simulink model "Octacopter_Model"  (R2025b)
settings: Solver=VariableStepAuto  StartTime=0.0  StopTime=10  RelTol=1e-3
values from neighbouring files (symbols this model uses):
  Alt = 600    [Octa_Initialise.m]
  c = -500    [Octa_Initialise.m]
  Drag_on = 1    [Octa_Initialise.m]
  g = 9.81    [Octa_Initialise.m]
  I = [I_xx, I_xy, I_xz; I_xy, I_yy, I_yz; I_xz, I_yz, I_zz]    [Octa_Initialise.m]
  I_xx = 0.35    [Octa_Initialise.m]
  I_yy = 0.35    [Octa_Initialise.m]
  I_zz = 0.67    [Octa_Initialise.m]
  k = 6500    [Octa_Initialise.m]
  k_D = [0.05, 0.05, 0.15]    [Octa_Initialise.m]
  k_q = (Cp*Rho*(D)^5)/(8*(pi)^3)    (= 1.08765022525e-07)    [Octa_Initialise.m]
  l_arm1 = [l*cosd(0) l*sind(0) 0]    [Octa_Initialise.m]
  l_arm2 = [l*cosd(-45) l*sind(-45) 0]    [Octa_Initialise.m]
  l_arm3 = [l*cosd(-90) l*sind(-90) 0]    [Octa_Initialise.m]
  l_arm4 = [l*cosd(-135) l*sind(-135) 0]    [Octa_Initialise.m]
  l_arm5 = [l*cosd(-180) l*sind(-180) 0]    [Octa_Initialise.m]
  l_arm6 = [l*cosd(135) l*sind(135) 0]    [Octa_Initialise.m]
  l_arm7 = [l*cosd(90) l*sind(90) 0]    [Octa_Initialise.m]
  l_arm8 = [l*cosd(45) l*sind(45) 0]    [Octa_Initialise.m]
  m = 6.71    [Octa_Initialise.m]
  M1_set_phi = 0    [Octa_Initialise.m]
  M1_set_theta = 0    [Octa_Initialise.m]
  M2_set_phi = 0    [Octa_Initialise.m]
  M2_set_theta = 0    [Octa_Initialise.m]
  M3_set_phi = 0    [Octa_Initialise.m]
  M3_set_theta = 0    [Octa_Initialise.m]
  M4_set_phi = 0    [Octa_Initialise.m]
  M4_set_theta = 0    [Octa_Initialise.m]
  M5_set_phi = 0    [Octa_Initialise.m]
  M5_set_theta = 0    [Octa_Initialise.m]
  M6_set_phi = 0    [Octa_Initialise.m]
  M6_set_theta = 0    [Octa_Initialise.m]
  M7_set_phi = 0    [Octa_Initialise.m]
  M7_set_theta = 0    [Octa_Initialise.m]
  M8_set_phi = 0    [Octa_Initialise.m]
  M8_set_theta = 0    [Octa_Initialise.m]
  p_dot_dot_0 = 0    [Octa_Initialise.m]
  phi_dot_0 = phi_theta_psi_dot_0(1)    [Octa_Initialise.m]
  phi_lower = deg2rad(-180)    [Octa_Initialise.m]
  phi_upper = deg2rad(180)    [Octa_Initialise.m]
  psi_dot_0 = phi_theta_psi_dot_0(3)    [Octa_Initialise.m]
  q_dot_dot_0 = 0    [Octa_Initialise.m]
  r_dot_dot_0 = 0    [Octa_Initialise.m]
  rpm2rad_s = pi/30    (= 0.10471975512)    [Octa_Initialise.m]
  RPM_max = 17668    [Octa_Initialise.m]    (also in Thrust_Plots.m = 15000)
  RPM_min = 0    [Octa_Initialise.m]    (also in Thrust_Plots.m)
  Tau_ESC1 = 0.15    [Octa_Initialise.m]
  Tau_ESC2 = 0.15    [Octa_Initialise.m]
  Tau_ESC3 = 0.15    [Octa_Initialise.m]
  Tau_ESC4 = 0.15    [Octa_Initialise.m]
  Tau_ESC5 = 0.15    [Octa_Initialise.m]
  Tau_ESC6 = 0.15    [Octa_Initialise.m]
  Tau_ESC7 = 0.15    [Octa_Initialise.m]
  Tau_ESC8 = 0.15    [Octa_Initialise.m]
  theta_dot_0 = phi_theta_psi_dot_0(2)    [Octa_Initialise.m]
  theta_lower = deg2rad(-90)    [Octa_Initialise.m]
  theta_upper = deg2rad(90)    [Octa_Initialise.m]
  Thrust_max = 20    [Octa_Initialise.m]
  thrustData = load('Cine66 Thrust Params.mat')    [Thrust_Plots.m]
  u_0 = u_v_w_0(1)    [Octa_Initialise.m]
  u_dot_0 = 0    [Octa_Initialise.m]
  v_0 = u_v_w_0(2)    [Octa_Initialise.m]
  v_dot_0 = 0    [Octa_Initialise.m]
  w1_0 = 0    [Octa_Initialise.m]
  w2_0 = 0    [Octa_Initialise.m]
  w3_0 = 0    [Octa_Initialise.m]
  w4_0 = 0    [Octa_Initialise.m]
  w5_0 = 0    [Octa_Initialise.m]
  w6_0 = 0    [Octa_Initialise.m]
  w7_0 = 0    [Octa_Initialise.m]
  w8_0 = 0    [Octa_Initialise.m]
  w_0 = u_v_w_0(3)    [Octa_Initialise.m]
  w_d_1 = -1    [Octa_Initialise.m]
  w_d_2 = +1.    (= 1)    [Octa_Initialise.m]
  w_d_3 = -1    [Octa_Initialise.m]
  w_d_4 = +1    (= 1)    [Octa_Initialise.m]
  w_d_5 = -1    [Octa_Initialise.m]
  w_d_6 = +1    (= 1)    [Octa_Initialise.m]
  w_d_7 = -1    [Octa_Initialise.m]
  w_d_8 = +1    (= 1)    [Octa_Initialise.m]
  w_dot_0 = 0    [Octa_Initialise.m]
undefined symbols (not defined in the file or in its folder): DiscIntNeverNeededParam
libraries: matrix_library x10, simulink x3, px4uORBlib x2, px4Sensorslib x2, sharedtransform x1, aerolibutil x1, px4Peripheralslib x1
(part 2 of 2)

== matlab function Octacopter_Model/Plant/Force & Moments/Thrust Forces and Moments/MATLAB Function10 ==
  data: phi input; theta input; T_mot_in input; T_b_out output
function T_b_out = fcn(phi, theta, T_mot_in)
%#codegen

%       phi    : phi angle (phi) about the body x-axis (radians)
%       theta   : theta angle (theta) about the intermediate y-axis (radians)
%       psi     : psi angle (psi) about the inertial z-axis (radians)
%
%   Note: This function assumes a standard Z-Y-X (psi-theta-phi) rotation
%   sequence to construct the rotation matrix R_i_b.

    % --- 1. Define the elementary rotation matrices ---
    
    % phi Rotation about x-axis (R_x(phi))
    Rx = [1,           0,          0;
          0,    cos(phi), -sin(phi);
          0,    sin(phi),  cos(phi)];
      
    % theta Rotation about y-axis (R_y(theta))
    Ry = [cos(theta),  0, sin(theta);
                 0,  1,          0;
         -sin(theta),  0, cos(theta)];
     

    % --- 2. Construct the full Rotation Matrix (DCM) ---
    % R_i_b = R_x(phi) * R_y(theta) 
    % This transforms a vector from  Inertial (i) to Body (b) frame.
    R_i_b = Rx * Ry;
    
    % --- 3. Apply the transformation ---
    T_b_out = R_i_b * T_mot_in;

== matlab function Octacopter_Model/Plant/Force & Moments/Thrust Forces and Moments/MATLAB Function11 ==
  data: phi input; theta input; T_mot_in input; T_b_out output
function T_b_out = fcn(phi, theta, T_mot_in)
%#codegen

%       phi    : phi angle (phi) about the body x-axis (radians)
%       theta   : theta angle (theta) about the intermediate y-axis (radians)
%       psi     : psi angle (psi) about the inertial z-axis (radians)
%
%   Note: This function assumes a standard Z-Y-X (psi-theta-phi) rotation
%   sequence to construct the rotation matrix R_i_b.

    % --- 1. Define the elementary rotation matrices ---
    
    % phi Rotation about x-axis (R_x(phi))
    Rx = [1,           0,          0;
          0,    cos(phi), -sin(phi);
          0,    sin(phi),  cos(phi)];
      
    % theta Rotation about y-axis (R_y(theta))
    Ry = [cos(theta),  0, sin(theta);
                 0,  1,          0;
         -sin(theta),  0, cos(theta)];
     

    % --- 2. Construct the full Rotation Matrix (DCM) ---
    % R_i_b = R_x(phi) * R_y(theta) 
    % This transforms a vector from  Inertial (i) to Body (b) frame.
    R_i_b = Rx * Ry;
    
    % --- 3. Apply the transformation ---
    T_b_out = R_i_b * T_mot_in;

== matlab function Octacopter_Model/Plant/Force & Moments/Thrust Forces and Moments/MATLAB Function12 ==
  data: phi input; theta input; T_mot_in input; T_b_out output
function T_b_out = fcn(phi, theta, T_mot_in)
%#codegen

%       phi    : phi angle (phi) about the body x-axis (radians)
%       theta   : theta angle (theta) about the intermediate y-axis (radians)
%       psi     : psi angle (psi) about the inertial z-axis (radians)
%
%   Note: This function assumes a standard Z-Y-X (psi-theta-phi) rotation
%   sequence to construct the rotation matrix R_i_b.

    % --- 1. Define the elementary rotation matrices ---
    
    % phi Rotation about x-axis (R_x(phi))
    Rx = [1,           0,          0;
          0,    cos(phi), -sin(phi);
          0,    sin(phi),  cos(phi)];
      
    % theta Rotation about y-axis (R_y(theta))
    Ry = [cos(theta),  0, sin(theta);
                 0,  1,          0;
         -sin(theta),  0, cos(theta)];
     

    % --- 2. Construct the full Rotation Matrix (DCM) ---
    % R_i_b = R_x(phi) * R_y(theta) 
    % This transforms a vector from  Inertial (i) to Body (b) frame.
    R_i_b = Rx * Ry;
    
    % --- 3. Apply the transformation ---
    T_b_out = R_i_b * T_mot_in;

== matlab function Octacopter_Model/Subsystem/Estimation1/MATLAB Function ==
  data: yaw_w input; yaw_u output
function yaw_u = unwrap_yaw(yaw_w)
% yaw_w: wrapped yaw [rad], typically in [-pi, pi]
% yaw_u: continuous yaw [rad]

persistent yaw_prev yaw_accum initialized

if isempty(initialized)
    yaw_prev = yaw_w;
    yaw_accum = yaw_w;
    initialized = true;
end

dyaw = yaw_w - yaw_prev;

% wrap increment to [-pi, pi]
dyaw = mod(dyaw + pi, 2*pi) - pi;

yaw_accum = yaw_accum + dyaw;
yaw_prev = yaw_w;

yaw_u = yaw_accum;

== matlab function Octacopter_Model/Plant/EOM/MATLAB Function ==
  data: phi input; PhiThetaPsi_dot output; theta input; pqr_dot input
function PhiThetaPsi_dot = fcn(phi, theta, pqr_dot)
%#codegen

Rot = [
    1 sind(phi)*tan(theta) cosd(phi)*tan(theta);
    0 cosd(theta) -sind(phi);
    0 sin(phi)*secd(theta) cosd(phi)*secd(theta)
    ];

PhiThetaPsi_dot = Rot*pqr_dot;

== matlab function Octacopter_Model/Plant/EOM/MATLAB Function1 ==
  data: F_b_net input; phi input; xyz_dot_dot output; theta input; psi input
function xyz_dot_dot = fcn(F_b_net, phi, theta, psi)
%#codegen
% BODY_TO_INERTIAL Converts a vector from the Body Frame to the Inertial Frame.
%
%   v_inertial = BODY_TO_INERTIAL(v_body, phi, theta, psi)
%
%   Inputs:
%       v_body  : 3x1 vector in the Body Frame (e.g., [x_b; y_b; z_b])
%       phi    : phi angle (phi) about the body x-axis (radians)
%       theta   : theta angle (theta) about the intermediate y-axis (radians)
%       psi     : psi angle (psi) about the inertial z-axis (radians)
%
%   Output:
%       v_inertial : 3x1 vector in the Inertial Frame (e.g., [x_i; y_i; z_i])
%
%   Note: This function assumes a standard Z-Y-X (psi-theta-phi) rotation
%   sequence to construct the rotation matrix R_i_b.

    % --- 1. Define the elementary rotation matrices ---
    
    % phi Rotation about x-axis (R_x(phi))
    Rx = [1,           0,          0;
          0,    cos(phi), -sin(phi);
          0,    sin(phi),  cos(phi)];
      
    % theta Rotation about y-axis (R_y(theta))
    Ry = [cos(theta),  0, sin(theta);
                 0,  1,          0;
         -sin(theta),  0, cos(theta)];
     
    % psi Rotation about z-axis (R_z(psi))
    Rz = [cos(psi), -sin(psi), 0;
          sin(psi),  cos(psi), 0;
               0,         0, 1];
    
    % --- 2. Construct the full Rotation Matrix (DCM) ---
    % R_i_b = R_x(phi) * R_y(theta) * R_z(psi)
    % This transforms a vector from Body (b) to Inertial (i) frame.
    R_i_b = Rz * Ry * Rx;
    
    % --- 3. Apply the transformation ---
    xyz_dot_dot = R_i_b * F_b_net;

== matlab function Octacopter_Model/Plant/EOM/MATLAB Function2 ==
  data: xyz_dot input; phi input; theta input; psi input; uvw output
function uvw = fcn( xyz_dot,phi, theta, psi)
%#codegen

%       phi    : phi angle (phi) about the body x-axis (radians)
%       theta   : theta angle (theta) about the intermediate y-axis (radians)
%       psi     : psi angle (psi) about the inertial z-axis (radians)
%
%   Note: This function assumes a standard Z-Y-X (psi-theta-phi) rotation
%   sequence to construct the rotation matrix R_i_b.

    % --- 1. Define the elementary rotation matrices ---
    
    % phi Rotation about x-axis (R_x(phi))
    Rx = [1,           0,          0;
          0,    cos(phi), -sin(phi);
          0,    sin(phi),  cos(phi)];
      
    % theta Rotation about y-axis (R_y(theta))
    Ry = [cos(theta),  0, sin(theta);
                 0,  1,          0;
         -sin(theta),  0, cos(theta)];
     
    % psi Rotation about z-axis (R_z(psi))
    Rz = [cos(psi), -sin(psi), 0;
          sin(psi),  cos(psi), 0;
               0,         0, 1];
    
    % --- 2. Construct the full Rotation Matrix (DCM) ---
    % R_i_b = R_x(phi) * R_y(theta) * R_z(psi)
    % This transforms a vector from  Inertial (i) to Body (b) frame.
    R_i_b = Rx * Ry * Rz;
    
    % --- 3. Apply the transformation ---
    uvw = R_i_b * xyz_dot;

== matlab function Octacopter_Model/Subsystem/motor mxer1 ==
  data: Roll input; M1 output; Pitch input; Thrust input; Yaw input; M2 output; M3 output; M4 output; M5 output; M6 output; M7 output; M8 output
function [M1, M2, M3, M4, M5, M6, M7, M8] = motor_mixer(Roll, Pitch, Thrust, Yaw)
% This function calculates motor commands for the 8-motor "plus" 
% configuration shown in your image.
%
% Inputs (assumed):
%   Roll, Pitch, Yaw: -1.0 to +1.0 control inputs
%   Thrust:             0.0 to 1.0 base throttle

% --- Configuration ---
idle_PWM = uint16(1000);
max_motor_val = single(1.0); % Max normalized output
min_motor_val = single(0.0); % Min normalized output

% This scaling method is from your example. It scales the control 
% inputs by the thrust level. You may need to tune the '4.0'
% denominator for best performance.
control_scale = Thrust / single(4.0);

% --- Mixer Logic ---
% Calculate normalized motor values (0.0 to 1.0 range) based on the diagram.
% We use single() to ensure floating-point math, as in your example.

% M1 (Front, CCW): -Pitch, +Yaw
m1_norm = ( ( -Pitch + Yaw ) * control_scale + Thrust );

% M2 (Back, CCW): +Pitch, +Yaw
m2_norm = ( (  Pitch + Yaw ) * control_scale + Thrust );

% M3 (Front-Right, CW): -Pitch, -Roll, -Yaw
m3_norm = ( ( -Pitch - Roll - Yaw ) * control_scale + Thrust );

% M4 (Back-Right, CW): +Pitch, -Roll, -Yaw
m4_norm = ( (  Pitch - Roll - Yaw ) * control_scale + Thrust );

% M5 (Front-Left, CW): -Pitch, +Roll, -Yaw
m5_norm = ( ( -Pitch + Roll - Yaw ) * control_scale + Thrust );

% M6 (Back-Left, CW): +Pitch, +Roll, -Yaw
m6_norm = ( (  Pitch + Roll - Yaw ) * control_scale + Thrust );

% M7 (Left, CCW): +Roll, +Yaw
m7_norm = ( (  Roll + Yaw ) * control_scale + Thrust );

% M8 (Right, CCW): -Roll, +Yaw
m8_norm = ( ( -Roll + Yaw ) * control_scale + Thrust );


% --- Output Scaling and Clamping ---
% It's CRITICAL to clamp (saturate) the motor commands between 0.0 and 1.0
% to prevent errors and ensure motor outputs are valid.
motors_norm = [m1_norm, m2_norm, m3_norm, m4_norm, m5_norm, m6_norm, m7_norm, m8_norm];
motors_norm = min(max(motors_norm, min_motor_val), max_motor_val);

% Convert normalized values (0.0-1.0) to PWM (1000-2000)
M1 = uint16(motors_norm(1) * single(1000)) + idle_PWM;
M2 = uint16(motors_norm(2) * single(1000)) + idle_PWM;
M3 = uint16(motors_norm(3) * single(1000)) + idle_PWM;
M4 = uint16(motors_norm(4) * single(1000)) + idle_PWM;
M5 = uint16(motors_norm(5) * single(1000)) + idle_PWM;
M6 = uint16(motors_norm(6) * single(1000)) + idle_PWM;
M7 = uint16(motors_norm(7) * single(1000)) + idle_PWM;
M8 = uint16(motors_norm(8) * single(1000)) + idle_PWM;

end

== matlab function Octacopter_Model/Plant/Force & Moments/Other Forces/Landing Gear Force/MATLAB Function3 ==
  data: phi input; theta input; psi input; F_b_Ldg output; F_ldg input
function F_b_Ldg = fcn(phi, theta, psi, F_ldg)
%#codegen

%       phi    : phi angle (phi) about the body x-axis (radians)
%       theta   : theta angle (theta) about the intermediate y-axis (radians)
%       psi     : psi angle (psi) about the inertial z-axis (radians)
%
%   Note: This function assumes a standard Z-Y-X (psi-theta-phi) rotation
%   sequence to construct the rotation matrix R_i_b.

    % --- 1. Define the elementary rotation matrices ---
    
    % phi Rotation about x-axis (R_x(phi))
    Rx = [1,           0,          0;
          0,    cos(phi), -sin(phi);
          0,    sin(phi),  cos(phi)];
      
    % theta Rotation about y-axis (R_y(theta))
    Ry = [cos(theta),  0, sin(theta);
                 0,  1,          0;
         -sin(theta),  0, cos(theta)];
     
    % psi Rotation about z-axis (R_z(psi))
    Rz = [cos(psi), -sin(psi), 0;
          sin(psi),  cos(psi), 0;
               0,         0, 1];
    
    % --- 2. Construct the full Rotation Matrix (DCM) ---
    % R_i_b = R_x(phi) * R_y(theta) * R_z(psi)
    % This transforms a vector from  Inertial (i) to Body (b) frame.
    R_i_b = Rx * Ry * Rz;
    
    % --- 3. Apply the transformation ---
    F_b_Ldg = R_i_b * F_ldg;

== matlab function Octacopter_Model/Plant/Force & Moments/Other Forces/Inertial 2 Body ==
  data: phi input; theta input; psi input; F_D_b output; F_D_i input
function F_D_b = fcn(phi, theta, psi, F_D_i)
%#codegen

%       phi    : phi angle (phi) about the body x-axis (radians)
%       theta   : theta angle (theta) about the intermediate y-axis (radians)
%       psi     : psi angle (psi) about the inertial z-axis (radians)
%
%   Note: This function assumes a standard Z-Y-X (psi-theta-phi) rotation
%   sequence to construct the rotation matrix R_i_b.

    % --- 1. Define the elementary rotation matrices ---
    
    % phi Rotation about x-axis (R_x(phi))
    Rx = [1,           0,          0;
          0,    cos(phi), -sin(phi);
          0,    sin(phi),  cos(phi)];
      
    % theta Rotation about y-axis (R_y(theta))
    Ry = [cos(theta),  0, sin(theta);
                 0,  1,          0;
         -sin(theta),  0, cos(theta)];
     
    % psi Rotation about z-axis (R_z(psi))
    Rz = [cos(psi), -sin(psi), 0;
          sin(psi),  cos(psi), 0;
               0,         0, 1];
    
    % --- 2. Construct the full Rotation Matrix (DCM) ---
    % R_i_b = R_x(phi) * R_y(theta) * R_z(psi)
    % This transforms a vector from  Inertial (i) to Body (b) frame.
    R_i_b = Rx * Ry * Rz;
    
    % --- 3. Apply the transformation ---
    F_D_b = R_i_b*F_D_i;

== matlab function Octacopter_Model/Plant/Force & Moments/Other Forces/Gravity Force ==
  data: phi input; theta input; psi input; F_g output; m_g input
function F_g = fcn(phi, theta, psi, m_g)
%#codegen

%       phi    : phi angle (phi) about the body x-axis (radians)
%       theta   : theta angle (theta) about the intermediate y-axis (radians)
%       psi     : psi angle (psi) about the inertial z-axis (radians)
%
%   Note: This function assumes a standard Z-Y-X (psi-theta-phi) rotation
%   sequence to construct the rotation matrix R_i_b.

    % --- 1. Define the elementary rotation matrices ---
    
    % phi Rotation about x-axis (R_x(phi))
    Rx = [1,           0,          0;
          0,    cos(phi), -sin(phi);
          0,    sin(phi),  cos(phi)];
      
    % theta Rotation about y-axis (R_y(theta))
    Ry = [cos(theta),  0, sin(theta);
                 0,  1,          0;
         -sin(theta),  0, cos(theta)];
     
    % psi Rotation about z-axis (R_z(psi))
    Rz = [cos(psi), -sin(psi), 0;
          sin(psi),  cos(psi), 0;
               0,         0, 1];
    
    % --- 2. Construct the full Rotation Matrix (DCM) ---
    % R_i_b = R_x(phi) * R_y(theta) * R_z(psi)
    % This transforms a vector from  Inertial (i) to Body (b) frame.
    R_i_b = Rx * Ry * Rz;
    
    % --- 3. Apply the transformation ---
    F_g = R_i_b * [0 0 -m_g]';

== matlab function Octacopter_Model/Plant/Force & Moments/Other Forces/Drag Force ==
  data: F_D output; u input; v input; w input; k_D input
function F_D = fcn(u, v, w, k_D)
%#codegen
    
    k_d_x = k_D(1);
    k_d_y = k_D(2);
    k_d_z = k_D(3);
    
    F_D_x = u*u*k_d_x;
    F_D_y = v*v*k_d_y;
    F_D_z = w*w*k_d_z;

    % --- 3. Apply the transformation ---
    F_D = [F_D_x; F_D_y; F_D_z;];

== matlab function Octacopter_Model/Plant/Force & Moments/Thrust Forces and Moments/MATLAB Function9 ==
  data: phi input; theta input; T_mot_in input; T_b_out output
function T_b_out = fcn(phi, theta, T_mot_in)
%#codegen

%       phi    : phi angle (phi) about the body x-axis (radians)
%       theta   : theta angle (theta) about the intermediate y-axis (radians)
%       psi     : psi angle (psi) about the inertial z-axis (radians)
%
%   Note: This function assumes a standard Z-Y-X (psi-theta-phi) rotation
%   sequence to construct the rotation matrix R_i_b.

    % --- 1. Define the elementary rotation matrices ---
    
    % phi Rotation about x-axis (R_x(phi))
    Rx = [1,           0,          0;
          0,    cos(phi), -sin(phi);
          0,    sin(phi),  cos(phi)];
      
    % theta Rotation about y-axis (R_y(theta))
    Ry = [cos(theta),  0, sin(theta);
                 0,  1,          0;
         -sin(theta),  0, cos(theta)];
     

    % --- 2. Construct the full Rotation Matrix (DCM) ---
    % R_i_b = R_x(phi) * R_y(theta) 
    % This transforms a vector from  Inertial (i) to Body (b) frame.
    R_i_b = Rx * Ry;
    
    % --- 3. Apply the transformation ---
    T_b_out = R_i_b * T_mot_in;

== matlab function Octacopter_Model/Plant/Force & Moments/Thrust Forces and Moments/MATLAB Function5 ==
  data: phi input; theta input; T_mot_in input; T_b_out output
function T_b_out = fcn(phi, theta, T_mot_in)
%#codegen

%       phi    : phi angle (phi) about the body x-axis (radians)
%       theta   : theta angle (theta) about the intermediate y-axis (radians)
%       psi     : psi angle (psi) about the inertial z-axis (radians)
%
%   Note: This function assumes a standard Z-Y-X (psi-theta-phi) rotation
%   sequence to construct the rotation matrix R_i_b.

    % --- 1. Define the elementary rotation matrices ---
    
    % phi Rotation about x-axis (R_x(phi))
    Rx = [1,           0,          0;
          0,    cos(phi), -sin(phi);
          0,    sin(phi),  cos(phi)];
      
    % theta Rotation about y-axis (R_y(theta))
    Ry = [cos(theta),  0, sin(theta);
                 0,  1,          0;
         -sin(theta),  0, cos(theta)];
     

    % --- 2. Construct the full Rotation Matrix (DCM) ---
    % R_i_b = R_x(phi) * R_y(theta) 
    % This transforms a vector from  Inertial (i) to Body (b) frame.
    R_i_b = Rx * Ry;
    
    % --- 3. Apply the transformation ---
    T_b_out = R_i_b * T_mot_in;

== matlab function Octacopter_Model/Plant/Force & Moments/Thrust Forces and Moments/MATLAB Function6 ==
  data: phi input; theta input; T_mot_in input; T_b_out output
function T_b_out = fcn(phi, theta, T_mot_in)
%#codegen

%       phi    : phi angle (phi) about the body x-axis (radians)
%       theta   : theta angle (theta) about the intermediate y-axis (radians)
%       psi     : psi angle (psi) about the inertial z-axis (radians)
%
%   Note: This function assumes a standard Z-Y-X (psi-theta-phi) rotation
%   sequence to construct the rotation matrix R_i_b.

    % --- 1. Define the elementary rotation matrices ---
    
    % phi Rotation about x-axis (R_x(phi))
    Rx = [1,           0,          0;
          0,    cos(phi), -sin(phi);
          0,    sin(phi),  cos(phi)];
      
    % theta Rotation about y-axis (R_y(theta))
    Ry = [cos(theta),  0, sin(theta);
                 0,  1,          0;
         -sin(theta),  0, cos(theta)];
     

    % --- 2. Construct the full Rotation Matrix (DCM) ---
    % R_i_b = R_x(phi) * R_y(theta) 
    % This transforms a vector from  Inertial (i) to Body (b) frame.
    R_i_b = Rx * Ry;
    
    % --- 3. Apply the transformation ---
    T_b_out = R_i_b * T_mot_in;

== matlab function Octacopter_Model/Plant/Force & Moments/Thrust Forces and Moments/MATLAB Function7 ==
  data: phi input; theta input; T_mot_in input; T_b_out output
function T_b_out = fcn(phi, theta, T_mot_in)
%#codegen

%       phi    : phi angle (phi) about the body x-axis (radians)
%       theta   : theta angle (theta) about the intermediate y-axis (radians)
%       psi     : psi angle (psi) about the inertial z-axis (radians)
%
%   Note: This function assumes a standard Z-Y-X (psi-theta-phi) rotation
%   sequence to construct the rotation matrix R_i_b.

    % --- 1. Define the elementary rotation matrices ---
    
    % phi Rotation about x-axis (R_x(phi))
    Rx = [1,           0,          0;
          0,    cos(phi), -sin(phi);
          0,    sin(phi),  cos(phi)];
      
    % theta Rotation about y-axis (R_y(theta))
    Ry = [cos(theta),  0, sin(theta);
                 0,  1,          0;
         -sin(theta),  0, cos(theta)];
     

    % --- 2. Construct the full Rotation Matrix (DCM) ---
    % R_i_b = R_x(phi) * R_y(theta) 
    % This transforms a vector from  Inertial (i) to Body (b) frame.
    R_i_b = Rx * Ry;
    
    % --- 3. Apply the transformation ---
    T_b_out = R_i_b * T_mot_in;

== matlab function Octacopter_Model/Plant/Force & Moments/Thrust Forces and Moments/MATLAB Function8 ==
  data: phi input; theta input; T_mot_in input; T_b_out output
function T_b_out = fcn(phi, theta, T_mot_in)
%#codegen

%       phi    : phi angle (phi) about the body x-axis (radians)
%       theta   : theta angle (theta) about the intermediate y-axis (radians)
%       psi     : psi angle (psi) about the inertial z-axis (radians)
%
%   Note: This function assumes a standard Z-Y-X (psi-theta-phi) rotation
%   sequence to construct the rotation matrix R_i_b.

    % --- 1. Define the elementary rotation matrices ---
    
    % phi Rotation about x-axis (R_x(phi))
    Rx = [1,           0,          0;
          0,    cos(phi), -sin(phi);
          0,    sin(phi),  cos(phi)];
      
    % theta Rotation about y-axis (R_y(theta))
    Ry = [cos(theta),  0, sin(theta);
                 0,  1,          0;
         -sin(theta),  0, cos(theta)];
     

    % --- 2. Construct the full Rotation Matrix (DCM) ---
    % R_i_b = R_x(phi) * R_y(theta) 
    % This transforms a vector from  Inertial (i) to Body (b) frame.
    R_i_b = Rx * Ry;
    
    % --- 3. Apply the transformation ---
    T_b_out = R_i_b * T_mot_in;
